simulink model "Bacs_Exp"  (R2018b)
settings: Solver=ode5  StartTime=0.0  StopTime=900  FixedStep=0.01  RelTol=1e-3  AbsTol=1e-6
values from neighbouring files (symbols this model uses):
  A = [-(C1*Alfa1*H10^(Alfa1-1))/S1  0  0 ... (first row only)    [init.m]
  B = [1/S1 0 0]'    [init.m]
  C = [0 0 1]    [init.m]
  H0 = [H10;H20;H30]    [init.m]
  H30 = 0.15    [init.m]
  L1 = place(A',C',PoleL1)'    [init.m]
  Q0 = C3*H30^Alfa3    (= 0.000130011411968)    [init.m]
undefined symbols (not defined in the file or in its folder): GetBias, GetPumpChar, GetScaleCoeff, TankBaseAddress
settings Model: SimulationMode=external  ExtModeTrigDuration=100000  ExtModeTrigLevel=0.400000  Creator=jims  LastModifiedBy=valletn
settings SolverCC: AutoScaleAbsTol=off
settings DataIOCC: ExternalInput=[]  InitialState=[]  MaxDataPoints=5000  SaveFormat=Array  SignalLoggingSaveFormat=ModelDataLogs  SaveOutput=off  SaveTime=off  SignalLoggingName=sigsOut
settings OptimizationCC: BooleanDataType=off  ExpressionDepthLimit=2147483647  InitFltsAndDblsToZero=on
settings DebuggingCC: SaveWithParameterizedLinksMsg=none  UnderspecifiedInitializationDetection=Classic  MergeDetectMultiDrivingBlocksExec=none  SignalResolutionControl=TryResolveAllWithWarning  MultiTaskDSMMsg=warning  MultiTaskCondExecSysMsg=none  IntegerOverflowMsg=none  FcnCallInpInsideContextMsg=warning  StateNameClashWarn=warning  SFUnexpectedBacktrackingDiag=warning  SFNoUnconditionalDefaultTransitionDiag=warning  SFExecutionAtInitializationDiag=none  IntegerSaturationMsg=none
settings ModelReferenceCC: PropagateSignalLabelsOutOfModel=off
settings SFSimCC: SimUseLocalCustomCode=off
settings RTWCC: SystemTargetFile=sldrt.tlc  TemplateMakefile=sldrt.tmf  Description=Simulink Desktop Real-Time  RTWUseLocalCustomCode=off  RTWCompilerOptimization=on
settings CodeAppCC: MaxIdLength=95  StateflowObjectComments=on
settings SimulinkDesktopRealTimeCC: TargetPreCompLibLocation=C:\Program Files\MATLAB\R2018b\toolbox\sldrt\lib\win64  TargetLangStandard=C89/C90 (ANSI)  SupportVariableSizeSignals=off  PreserveStateflowLocalDataDimensions=off
settings ConfigComp: CovMetricSettings=dw  CovHtmlReporting=on  CovSaveCumulativeToWorkspaceVar=on  CovSaveSingleToWorkspaceVar=on  CovExternalEMLEnable=off

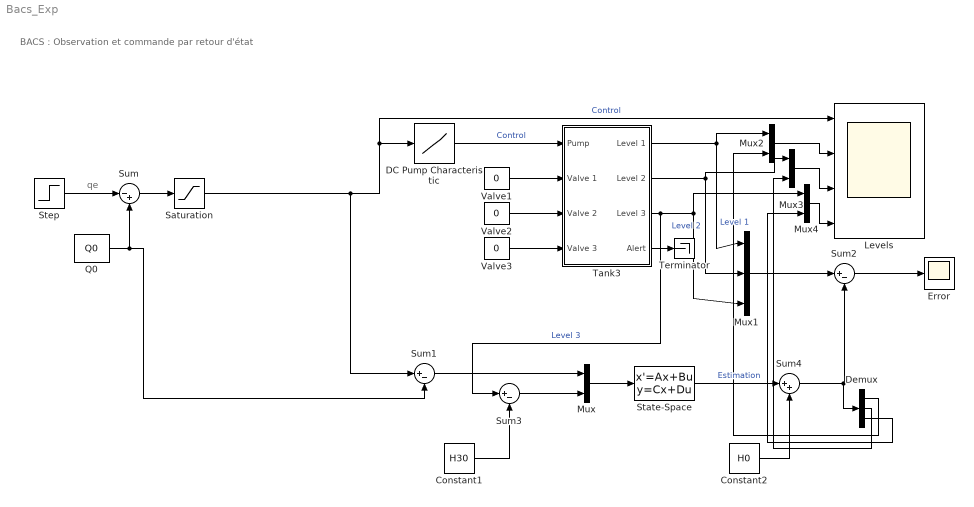
== system Bacs_Exp ==
  note: qe
  note: BACS : Observation et commande par retour d'état
  Constant1 : Constant  Value=H30
  Constant2 : Constant  Value=H0
  DC Pump Characteristic : Lookup  InputValues=GetPumpChar('Volume')  Table=GetPumpChar('control')  SaturateOnIntegerOverflow=on
  Demux : Demux  Outputs=3
  Error : Scope
  Levels : Scope  NumInputPorts=4
  Mux{,2..4} (4 alike) : Mux  Inputs=2
  Mux1 : Mux  Inputs=3
  Q0 : Constant  Value=Q0
  Saturation : Saturate  UpperLimit=GetPumpChar('MaxVolume')  LowerLimit=0
  State-Space : StateSpace  A=A-L1*C  B=[B L1]  C=eye(3)  D=zeros(3,2)  InitialCondition=0
  Step : Step  Time=300  After=0.1*Q0  SampleTime=0
  Sum : Sum  Inputs=|-+
  Sum1 : Sum  Inputs=|+-
  Sum2 : Sum  Inputs=|+-
  Sum3 : Sum  Inputs=|+-
  Sum4 : Sum  Inputs=|++
  Tank3 : Subsystem  mask{BaseAddress=TankBaseAddress, T0=0.01}
      mask prompts: BaseAddress "Base Address:"; T0 "Sampling Period:"
      mask Display: image(imread('MultiTank.bmp'))
  Terminator : Terminator
  Valve1 : Constant  Value=0
  Valve2 : Constant  Value=0
  Valve3 : Constant  Value=0
  wires:
  Valve3/1 -> Tank3/4(Valve 3)
  Saturation/1 -> Sum1/1, Levels/1, DC Pump Characteristic/1  "Control"
  Valve2/1 -> Tank3/3(Valve 2)
  Valve1/1 -> Tank3/2(Valve 1)
  Tank3/4(Alert) -> Terminator/1
  DC Pump Characteristic/1 -> Tank3/1(Pump)  "Control"
  Tank3/1(Level 1) -> Mux1/1, Mux2/1  "Level 1"
  Tank3/2(Level 2) -> Mux1/2, Mux3/1  "Level 2"
  Tank3/3(Level 3) -> Sum3/1, Mux1/3, Mux4/1  "Level 3"
  Q0/1 -> Sum1/2, Sum/2
  Sum/1 -> Saturation/1
  Step/1 -> Sum/1
  Sum3/1 -> Mux/2
  State-Space/1 -> Sum4/1  "Estimation"
  Sum1/1 -> Mux/1
  Mux/1 -> State-Space/1
  Constant2/1 -> Sum4/2
  Constant1/1 -> Sum3/2
  Sum4/1 -> Demux/1, Sum2/2
  Sum2/1 -> Error/1
  Mux1/1 -> Sum2/1
  Mux2/1 -> Levels/2
  Demux/1 -> Mux2/2
  Mux3/1 -> Levels/3
  Demux/2 -> Mux3/2
  Mux4/1 -> Levels/4
  Demux/3 -> Mux4/2

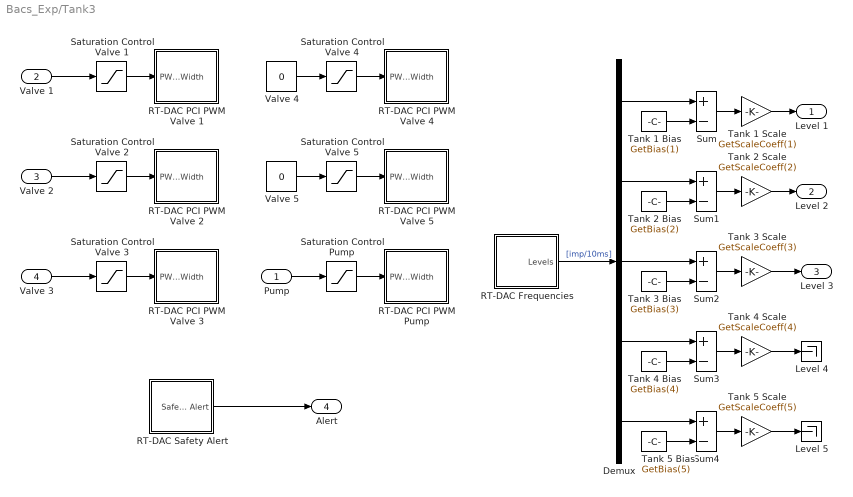
== system Bacs_Exp/Tank3 ==
  Pump : Inport
  Valve 1 : Inport  Port=2
  Valve 2 : Inport  Port=3
  Valve 3 : Inport  Port=4
  Demux : Demux  Outputs=5
  Level 4 : Terminator
  Level 5 : Terminator
  RT-DAC Frequencies : Subsystem  mask(Analog Input Module){BaseAddress=BaseAddress, T0=T0}
      mask prompts: BaseAddress "Base Address:"; T0 "Sample Time (sec):"
      mask help: RT-DAC PCI Device Driver
      mask Help: Set up each field for your specific hardware configuration.
      mask Display: plot(0,0,100,100,[90,80,80,11,11],[90,90,20,20,80],[11,80],[80,80],[80,80],[20,14],[80,85,85,80],[45,45,66,66],[45,45,74,74],[20,13,13,20],[15,27,27,15,15],[75,75,26,26,75],[33,48,48,33,33],[75,75,55,55,75],[55,55,71,71,55],[55,75,75,55,55],[33,41,41,33,33],[50,50,27,27,50],[48,56,56,48,48],[50,50,27,27,50],[62,70,70,62,62],[50,50,27,27,50])
  RT-DAC Safety Alert : Subsystem  mask(Analog Input Module){BaseAddress=BaseAddress, T0=T0}
      mask prompts: BaseAddress "Base Address:"; T0 "Sample Time (sec):"
      mask help: RT-DAC PCI Device Driver
      mask Help: Set up each field for your specific hardware configuration.
      mask Display: plot(0,0,100,100,[90,80,80,11,11],[90,90,20,20,80],[11,80],[80,80],[80,80],[20,14],[80,85,85,80],[45,45,66,66],[45,45,74,74],[20,13,13,20],[15,27,27,15,15],[75,75,26,26,75],[33,48,48,33,33],[75,75,55,55,75],[55,55,71,71,55],[55,75,75,55,55],[33,41,41,33,33],[50,50,27,27,50],[48,56,56,48,48],[50,50,27,27,50],[62,70,70,62,62],[50,50,27,27,50])
  RT-DAC PCI PWM Pump : Subsystem  mask(PWM Module){BaseAddress=BaseAddress, ChanIdx=0, ChanMode=12 Bit, ChanPresc=1, SetOutputsFlag=on, SetOutputsValue=0, T0=T0}
      mask prompts: BaseAddress "IO Base Address:"; ChanIdx "Channel:"; ChanMode "Channel Mode:"; ChanPresc "Channel Prescaler:"; SetOutputsFlag "Set Outputs At Termination"; SetOutputsValue "Termination Outputs:"; T0 "Sample Time (sec):"
      mask help: RT-DAC PCI Device Driver
      mask Help: Set up each field for your specific hardware configuration.
      mask TypeOptions ChanIdx: 0 | 1 | 2 | 3 | 4 | 5
      mask TypeOptions ChanMode: 8 Bit | 12 Bit
      mask Display: plot(0,0,100,100,[90,80,80,11,11],[90,90,20,20,80],[11,80],[80,80],[80,80],[20,14],[80,85,85,80],[45,45,66,66],[45,45,74,74],[20,13,13,20],[15,27,27,15,15],[75,75,26,26,75],[33,48,48,33,33],[75,75,55,55,75],[55,55,71,71,55],[55,75,75,55,55],[33,41,41,33,33],[50,50,27,27,50],[48,56,56,48,48],[50,50,27,27,50],[62,70,70,62,62],[50,50,27,27,50])
  RT-DAC PCI PWM Valve 1 : Subsystem  mask(PWM Module){BaseAddress=BaseAddress, ChanIdx=3, ChanMode=12 Bit, ChanPresc=31, SetOutputsFlag=on, SetOutputsValue=0, T0=T0}
      mask prompts: BaseAddress "IO Base Address:"; ChanIdx "Channel:"; ChanMode "Channel Mode:"; ChanPresc "Channel Prescaler:"; SetOutputsFlag "Set Outputs At Termination"; SetOutputsValue "Termination Outputs:"; T0 "Sample Time (sec):"
      mask help: RT-DAC PCI Device Driver
      mask Help: Set up each field for your specific hardware configuration.
      mask TypeOptions ChanIdx: 0 | 1 | 2 | 3 | 4 | 5
      mask TypeOptions ChanMode: 8 Bit | 12 Bit
      mask Display: plot(0,0,100,100,[90,80,80,11,11],[90,90,20,20,80],[11,80],[80,80],[80,80],[20,14],[80,85,85,80],[45,45,66,66],[45,45,74,74],[20,13,13,20],[15,27,27,15,15],[75,75,26,26,75],[33,48,48,33,33],[75,75,55,55,75],[55,55,71,71,55],[55,75,75,55,55],[33,41,41,33,33],[50,50,27,27,50],[48,56,56,48,48],[50,50,27,27,50],[62,70,70,62,62],[50,50,27,27,50])
  RT-DAC PCI PWM Valve 2 : Subsystem  mask(PWM Module){BaseAddress=BaseAddress, ChanIdx=2, ChanMode=12 Bit, ChanPresc=31, SetOutputsFlag=on, SetOutputsValue=0, T0=T0}
      mask prompts: BaseAddress "IO Base Address:"; ChanIdx "Channel:"; ChanMode "Channel Mode:"; ChanPresc "Channel Prescaler:"; SetOutputsFlag "Set Outputs At Termination"; SetOutputsValue "Termination Outputs:"; T0 "Sample Time (sec):"
      mask help: RT-DAC PCI Device Driver
      mask Help: Set up each field for your specific hardware configuration.
      mask TypeOptions ChanIdx: 0 | 1 | 2 | 3 | 4 | 5
      mask TypeOptions ChanMode: 8 Bit | 12 Bit
      mask Display: plot(0,0,100,100,[90,80,80,11,11],[90,90,20,20,80],[11,80],[80,80],[80,80],[20,14],[80,85,85,80],[45,45,66,66],[45,45,74,74],[20,13,13,20],[15,27,27,15,15],[75,75,26,26,75],[33,48,48,33,33],[75,75,55,55,75],[55,55,71,71,55],[55,75,75,55,55],[33,41,41,33,33],[50,50,27,27,50],[48,56,56,48,48],[50,50,27,27,50],[62,70,70,62,62],[50,50,27,27,50])
  RT-DAC PCI PWM Valve 3 : Subsystem  mask(PWM Module){BaseAddress=BaseAddress, ChanIdx=1, ChanMode=12 Bit, ChanPresc=31, SetOutputsFlag=on, SetOutputsValue=0, T0=T0}
      mask prompts: BaseAddress "IO Base Address:"; ChanIdx "Channel:"; ChanMode "Channel Mode:"; ChanPresc "Channel Prescaler:"; SetOutputsFlag "Set Outputs At Termination"; SetOutputsValue "Termination Outputs:"; T0 "Sample Time (sec):"
      mask help: RT-DAC PCI Device Driver
      mask Help: Set up each field for your specific hardware configuration.
      mask TypeOptions ChanIdx: 0 | 1 | 2 | 3 | 4 | 5
      mask TypeOptions ChanMode: 8 Bit | 12 Bit
      mask Display: plot(0,0,100,100,[90,80,80,11,11],[90,90,20,20,80],[11,80],[80,80],[80,80],[20,14],[80,85,85,80],[45,45,66,66],[45,45,74,74],[20,13,13,20],[15,27,27,15,15],[75,75,26,26,75],[33,48,48,33,33],[75,75,55,55,75],[55,55,71,71,55],[55,75,75,55,55],[33,41,41,33,33],[50,50,27,27,50],[48,56,56,48,48],[50,50,27,27,50],[62,70,70,62,62],[50,50,27,27,50])
  RT-DAC PCI PWM Valve 4 : Subsystem  mask(PWM Module){BaseAddress=BaseAddress, ChanIdx=5, ChanMode=12 Bit, ChanPresc=31, SetOutputsFlag=on, SetOutputsValue=0, T0=T0}
      mask prompts: BaseAddress "IO Base Address:"; ChanIdx "Channel:"; ChanMode "Channel Mode:"; ChanPresc "Channel Prescaler:"; SetOutputsFlag "Set Outputs At Termination"; SetOutputsValue "Termination Outputs:"; T0 "Sample Time (sec):"
      mask help: RT-DAC PCI Device Driver
      mask Help: Set up each field for your specific hardware configuration.
      mask TypeOptions ChanIdx: 0 | 1 | 2 | 3 | 4 | 5
      mask TypeOptions ChanMode: 8 Bit | 12 Bit
      mask Display: plot(0,0,100,100,[90,80,80,11,11],[90,90,20,20,80],[11,80],[80,80],[80,80],[20,14],[80,85,85,80],[45,45,66,66],[45,45,74,74],[20,13,13,20],[15,27,27,15,15],[75,75,26,26,75],[33,48,48,33,33],[75,75,55,55,75],[55,55,71,71,55],[55,75,75,55,55],[33,41,41,33,33],[50,50,27,27,50],[48,56,56,48,48],[50,50,27,27,50],[62,70,70,62,62],[50,50,27,27,50])
  RT-DAC PCI PWM Valve 5 : Subsystem  mask(PWM Module){BaseAddress=BaseAddress, ChanIdx=4, ChanMode=12 Bit, ChanPresc=31, SetOutputsFlag=on, SetOutputsValue=0, T0=T0}
      mask prompts: BaseAddress "IO Base Address:"; ChanIdx "Channel:"; ChanMode "Channel Mode:"; ChanPresc "Channel Prescaler:"; SetOutputsFlag "Set Outputs At Termination"; SetOutputsValue "Termination Outputs:"; T0 "Sample Time (sec):"
      mask help: RT-DAC PCI Device Driver
      mask Help: Set up each field for your specific hardware configuration.
      mask TypeOptions ChanIdx: 0 | 1 | 2 | 3 | 4 | 5
      mask TypeOptions ChanMode: 8 Bit | 12 Bit
      mask Display: plot(0,0,100,100,[90,80,80,11,11],[90,90,20,20,80],[11,80],[80,80],[80,80],[20,14],[80,85,85,80],[45,45,66,66],[45,45,74,74],[20,13,13,20],[15,27,27,15,15],[75,75,26,26,75],[33,48,48,33,33],[75,75,55,55,75],[55,55,71,71,55],[55,75,75,55,55],[33,41,41,33,33],[50,50,27,27,50],[48,56,56,48,48],[50,50,27,27,50],[62,70,70,62,62],[50,50,27,27,50])
  Saturation Control Pump : Saturate  UpperLimit=1  LowerLimit=0
  Saturation Control Valve {1..5} (5 alike) : Saturate  UpperLimit=1  LowerLimit=0
  Sum{,1..4} (5 alike) : Sum  Inputs=+-  SaturateOnIntegerOverflow=on  InputSameDT=on  OutDataTypeStr=Inherit: Same as first input
  Tank 1 Bias : Constant  Value=GetBias(1)
  Tank 1 Scale : Gain  Gain=GetScaleCoeff(1)  SaturateOnIntegerOverflow=on  OutDataTypeStr=Inherit: Same as input  ParamDataTypeStr=Inherit: Same as input
  Tank 2 Bias : Constant  Value=GetBias(2)
  Tank 2 Scale : Gain  Gain=GetScaleCoeff(2)  SaturateOnIntegerOverflow=on  OutDataTypeStr=Inherit: Same as input  ParamDataTypeStr=Inherit: Same as input
  Tank 3 Bias : Constant  Value=GetBias(3)
  Tank 3 Scale : Gain  Gain=GetScaleCoeff(3)  SaturateOnIntegerOverflow=on  OutDataTypeStr=Inherit: Same as input  ParamDataTypeStr=Inherit: Same as input
  Tank 4 Bias : Constant  Value=GetBias(4)
  Tank 4 Scale : Gain  Gain=GetScaleCoeff(4)  SaturateOnIntegerOverflow=on  OutDataTypeStr=Inherit: Same as input  ParamDataTypeStr=Inherit: Same as input
  Tank 5 Bias : Constant  Value=GetBias(5)
  Tank 5 Scale : Gain  Gain=GetScaleCoeff(5)  SaturateOnIntegerOverflow=on  OutDataTypeStr=Inherit: Same as input  ParamDataTypeStr=Inherit: Same as input
  Valve 4 : Constant  Value=0
  Valve 5 : Constant  Value=0
  Level 1 : Outport
  Level 2 : Outport  Port=2
  Level 3 : Outport  Port=3
  Alert : Outport  Port=4
  wires:
  Valve 1/1 -> Saturation Control Valve 1/1
  Saturation Control Valve 1/1 -> RT-DAC PCI PWM Valve 1/1(PWM Width)
  Saturation Control Valve 2/1 -> RT-DAC PCI PWM Valve 2/1(PWM Width)
  Saturation Control Valve 3/1 -> RT-DAC PCI PWM Valve 3/1(PWM Width)
  Saturation Control Valve 4/1 -> RT-DAC PCI PWM Valve 4/1(PWM Width)
  Saturation Control Valve 5/1 -> RT-DAC PCI PWM Valve 5/1(PWM Width)
  Saturation Control Pump/1 -> RT-DAC PCI PWM Pump/1(PWM Width)
  Pump/1 -> Saturation Control Pump/1
  Valve 2/1 -> Saturation Control Valve 2/1
  Valve 3/1 -> Saturation Control Valve 3/1
  Valve 4/1 -> Saturation Control Valve 4/1
  Valve 5/1 -> Saturation Control Valve 5/1
  RT-DAC Frequencies/1(Levels) -> Demux/1  "[imp/10ms]"
  Demux/1 -> Sum/1
  Demux/2 -> Sum1/1
  Demux/3 -> Sum2/1
  Demux/4 -> Sum3/1
  Demux/5 -> Sum4/1
  Sum/1 -> Tank 1 Scale/1
  Tank 1 Bias/1 -> Sum/2
  Sum1/1 -> Tank 2 Scale/1
  Tank 2 Bias/1 -> Sum1/2
  Tank 3 Bias/1 -> Sum2/2
  Sum2/1 -> Tank 3 Scale/1
  Tank 4 Bias/1 -> Sum3/2
  Tank 5 Bias/1 -> Sum4/2
  Sum4/1 -> Tank 5 Scale/1
  Sum3/1 -> Tank 4 Scale/1
  RT-DAC Safety Alert/1(Safety Alert) -> Alert/1
  Tank 1 Scale/1 -> Level 1/1
  Tank 2 Scale/1 -> Level 2/1
  Tank 3 Scale/1 -> Level 3/1
  Tank 4 Scale/1 -> Level 4/1
  Tank 5 Scale/1 -> Level 5/1

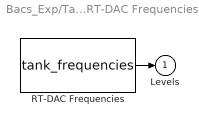
== system Bacs_Exp/Tank3/RT-DAC Frequencies ==
  RT-DAC Frequencies : S-Function  FunctionName=tank_frequencies  Parameters=BaseAddress, T0  SFunctionDeploymentMode=off  EnableBusSupport=off
  Levels : Outport
  wires:
  RT-DAC Frequencies/1 -> Levels/1

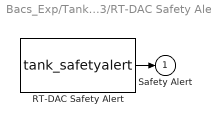
== system Bacs_Exp/Tank3/RT-DAC Safety Alert ==
  RT-DAC Safety Alert : S-Function  FunctionName=tank_safetyalert  Parameters=BaseAddress, T0  SFunctionDeploymentMode=off  EnableBusSupport=off
  Safety Alert : Outport
  wires:
  RT-DAC Safety Alert/1 -> Safety Alert/1

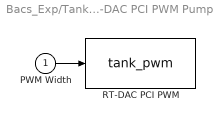
== system Bacs_Exp/Tank3/RT-DAC PCI PWM Pump ==
  PWM Width : Inport
  "RT-DAC PCI PWM " : S-Function  FunctionName=tank_pwm  Parameters=BaseAddress, ChanIdx, ChanMode, ChanPresc, SetOutputsFlag, SetOutputsValue, T0  SFunctionDeploymentMode=off  EnableBusSupport=off
  wires:
  PWM Width/1 -> "RT-DAC PCI PWM "/1

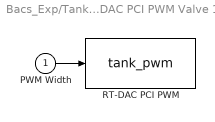
== system Bacs_Exp/Tank3/RT-DAC PCI PWM Valve 1 ==
  PWM Width : Inport
  "RT-DAC PCI PWM " : S-Function  FunctionName=tank_pwm  Parameters=BaseAddress, ChanIdx, ChanMode, ChanPresc, SetOutputsFlag, SetOutputsValue, T0  SFunctionDeploymentMode=off  EnableBusSupport=off
  wires:
  PWM Width/1 -> "RT-DAC PCI PWM "/1

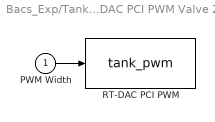
== system Bacs_Exp/Tank3/RT-DAC PCI PWM Valve 2 ==
  PWM Width : Inport
  "RT-DAC PCI PWM " : S-Function  FunctionName=tank_pwm  Parameters=BaseAddress, ChanIdx, ChanMode, ChanPresc, SetOutputsFlag, SetOutputsValue, T0  SFunctionDeploymentMode=off  EnableBusSupport=off
  wires:
  PWM Width/1 -> "RT-DAC PCI PWM "/1

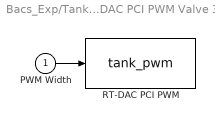
== system Bacs_Exp/Tank3/RT-DAC PCI PWM Valve 3 ==
  PWM Width : Inport
  "RT-DAC PCI PWM " : S-Function  FunctionName=tank_pwm  Parameters=BaseAddress, ChanIdx, ChanMode, ChanPresc, SetOutputsFlag, SetOutputsValue, T0  SFunctionDeploymentMode=off  EnableBusSupport=off
  wires:
  PWM Width/1 -> "RT-DAC PCI PWM "/1

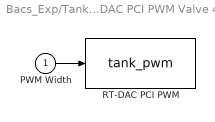
== system Bacs_Exp/Tank3/RT-DAC PCI PWM Valve 4 ==
  PWM Width : Inport
  "RT-DAC PCI PWM " : S-Function  FunctionName=tank_pwm  Parameters=BaseAddress, ChanIdx, ChanMode, ChanPresc, SetOutputsFlag, SetOutputsValue, T0  SFunctionDeploymentMode=off  EnableBusSupport=off
  wires:
  PWM Width/1 -> "RT-DAC PCI PWM "/1

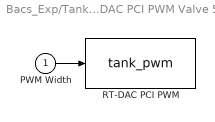
== system Bacs_Exp/Tank3/RT-DAC PCI PWM Valve 5 ==
  PWM Width : Inport
  "RT-DAC PCI PWM " : S-Function  FunctionName=tank_pwm  Parameters=BaseAddress, ChanIdx, ChanMode, ChanPresc, SetOutputsFlag, SetOutputsValue, T0  SFunctionDeploymentMode=off  EnableBusSupport=off
  wires:
  PWM Width/1 -> "RT-DAC PCI PWM "/1
